simulink model "sampleModel1430"  (R2023a)
settings: Solver=VariableStepAuto  StartTime=0.0  StopTime=10.0  RelTol=1e-3
libraries: hdlsllib x6, simulink x2
settings Model: Creator=user1  LastModifiedBy=user1

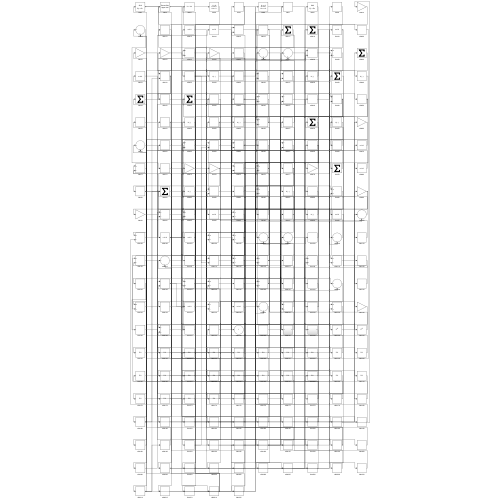
[thumbnail: Simulink's stored preview of the top-level diagram]
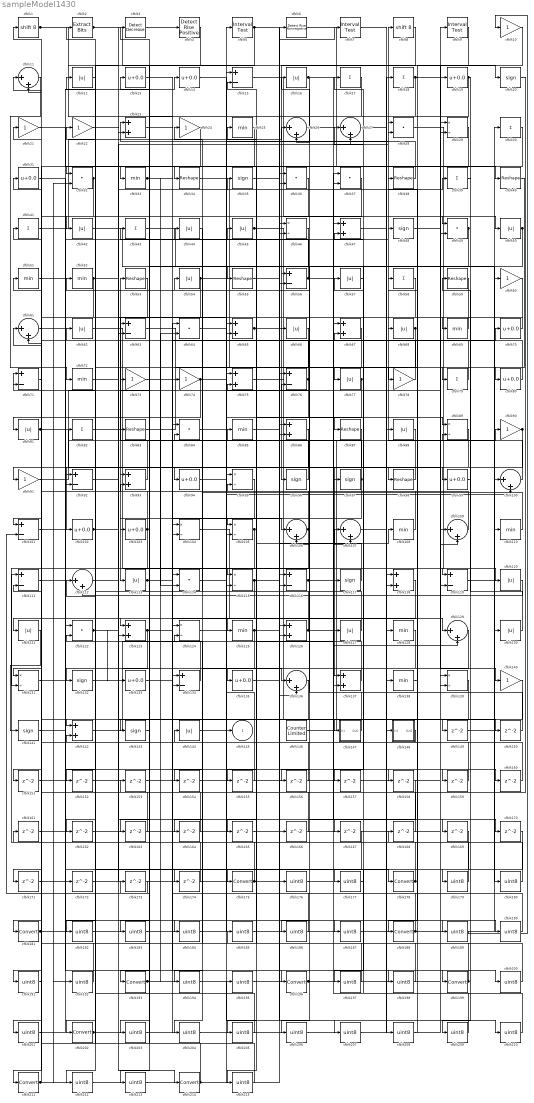
== system sampleModel1430 ==
  cfblk1 : ArithShift  BitShiftNumber=8
  cfblk{10,21..22,24,60,73..74,78,90..91,140} (11 alike) : Gain
  cfblk{11,26..27,61,100,106..107,109,112,129,136} (11 alike) : Sum  Inputs=|++
  cfblk{15,56,63,71,76,92,101,111,116,119,134} (11 alike) : Sum  Inputs=+-
  cfblk{13..14,19,31,70,80,94,99,102..103,133,135} (12 alike) : Bias  Bias=0.0  SaturateOnIntegerOverflow=off
  cfblk{29,46,89,95,104..105,115,124,131,139} (10 alike) : Product  Inputs=*/  RndMeth=Zero  SaturateOnIntegerOverflow=on
  cfblk{25,33,51..52,69,72,85,108,110,125,128,138} (12 alike) : MinMax
  cfblk{12,16,42,44..45,50,54,57,62,66,68,77,81,88,113,120..121,127,130,144} (20 alike) : Abs  SaturateOnIntegerOverflow=off
  cfblk{28,32,36..37,49,64,84,114,122} (9 alike) : DotProduct  OutDataTypeStr=Inherit: Inherit via internal rule
  cfblk{20,35,48,96..97,117,132,141,143} (9 alike) : Signum
  cfblk{23,47,65,67,75,86,93,118,123,126,137,142} (12 alike) : Sum
  cfblk146 : hdlsllib/Sources/Counter Limited  uplimit=7  tsamp=-1
  cfblk147 : Subsystem
      settings: LibrarySourceBlock=|
      | hdlsllib/Ports &
      | Subsystems/Subsystem
  cfblk148 : Subsystem
      settings: LibrarySourceBlock=|
      | hdlsllib/Ports &
      | Subsystems/Subsystem
  cfblk{149..174} (26 alike) : Delay  SampleTime=1
  cfblk{17..18,30,39,41,43,58,79,82} (9 alike) : Sum  Inputs=+
  cfblk{175,178,181,188,193,196,199,202,211,214} (10 alike) : DataTypeConversion  SaturateOnIntegerOverflow=off  RndMeth=Floor
  cfblk{176..177,179..180,182..187,189..192,194..195,197..198,200..201,203..210,212..213,215} (31 alike) : DataTypeConversion  OutDataTypeStr=uint8  SaturateOnIntegerOverflow=off  RndMeth=Floor
  cfblk2 : simulink/Logic and Bit Operations/Extract Bits  bitsToExtract=Upper half  numBits=8  bitIdxRange=[0 7]  outScalingMode=Preserve fixed-point scaling
      settings: LibrarySourceBlock=|
      | hdlsllib/Logic and Bit
      | Operations/Extract Bits
  cfblk3 : simulink/Logic and Bit Operations/Detect Decrease  vinit=0.0  OutDataTypeStr=boolean
      settings: LibrarySourceBlock=|
      | hdlsllib/Logic and Bit
      | Operations/Detect
      | Decrease
  cfblk{34,38,40,53,55,59,83,87,98} (9 alike) : Reshape
  cfblk4 : hdlsllib/Logic and Bit Operations/Detect Rise Positive  vinit=0  OutDataTypeStr=boolean
  cfblk5 : hdlsllib/Logic and Bit Operations/Interval Test  IntervalClosedRight=on  uplimit=0.5  IntervalClosedLeft=on  lowlimit=-0.5  OutDataTypeStr=boolean
  cfblk6 : hdlsllib/Logic and Bit Operations/Detect Rise Nonnegative  vinit=0  OutDataTypeStr=boolean
  cfblk7 : hdlsllib/Logic and Bit Operations/Interval Test  IntervalClosedRight=on  uplimit=0.5  IntervalClosedLeft=on  lowlimit=-0.5  OutDataTypeStr=boolean
  cfblk8 : ArithShift  BitShiftNumber=8
  cfblk9 : hdlsllib/Logic and Bit Operations/Interval Test  IntervalClosedRight=on  uplimit=0.5  IntervalClosedLeft=on  lowlimit=-0.5  OutDataTypeStr=boolean
  cfblk145 : Outport  VectorParamsAs1DForOutWhenUnconnected=off
  wires:
  cfblk146/1 -> cfblk90/1
  cfblk50/1 -> cfblk156/1, cfblk157/1
  cfblk25/1 -> cfblk34/1
  cfblk62/1 -> cfblk119/1
  cfblk75/1 -> cfblk147/1(In1)
  cfblk97/1 -> cfblk85/1, cfblk134/2
  cfblk83/1 -> cfblk77/1
  cfblk33/1 -> cfblk129/1, cfblk114/2, cfblk187/1
  cfblk28/1 -> cfblk120/1
  cfblk40/1 -> cfblk80/1
  cfblk130/1 -> cfblk59/1
  cfblk100/1 -> cfblk8/1
  cfblk123/1 -> cfblk142/1, cfblk89/2, cfblk150/1
  cfblk88/1 -> cfblk137/1
  cfblk45/1 -> cfblk98/1, cfblk28/2
  cfblk3/1 -> cfblk4/1
  cfblk102/1 -> cfblk27/2, cfblk76/2, cfblk184/1
  cfblk52/1 -> cfblk121/1, cfblk189/1
  cfblk8/1 -> cfblk96/1
  cfblk78/1 -> cfblk54/1
  cfblk15/1 -> cfblk50/1
  cfblk92/1 -> cfblk199/1
  cfblk104/1 -> cfblk127/1
  cfblk67/1 -> cfblk175/1
  cfblk93/1 -> cfblk53/1
  cfblk122/1 -> cfblk133/1, cfblk149/1
  cfblk139/1 -> cfblk202/1
  cfblk41/1 -> cfblk26/1
  cfblk82/1 -> cfblk113/1
  cfblk30/1 -> cfblk181/1
  cfblk11/1 -> cfblk72/1
  cfblk56/1 -> cfblk43/1, cfblk169/1
  cfblk114/1 -> cfblk5/1
  cfblk89/1 -> cfblk102/1
  cfblk49/1 -> cfblk105/1, cfblk137/2, cfblk56/1
  cfblk116/1 -> cfblk16/1, cfblk129/2
  cfblk79/1 -> cfblk31/1
  cfblk1/1 -> cfblk104/1, cfblk23/2
  cfblk98/1 -> cfblk94/1
  cfblk77/1 -> cfblk115/1, cfblk106/2
  cfblk34/1 -> cfblk110/1
  cfblk70/1 -> cfblk69/1
  cfblk138/1 -> cfblk38/1
  cfblk64/1 -> cfblk145/1
  cfblk59/1 -> cfblk93/1
  cfblk108/1 -> cfblk57/1
  cfblk134/1 -> cfblk62/1
  cfblk27/1 -> cfblk88/1
  cfblk19/1 -> cfblk103/1, cfblk99/1
  cfblk55/1 -> cfblk6/1
  cfblk54/1 -> cfblk203/1, cfblk210/1
  cfblk7/1 -> cfblk49/1
  cfblk147/1(Out1) -> cfblk52/1
  cfblk125/1 -> cfblk108/1, cfblk164/1
  cfblk9/1 -> cfblk119/2
  cfblk43/1 -> cfblk130/1
  cfblk111/1 -> cfblk178/1
  cfblk37/1 -> cfblk193/1
  cfblk103/1 -> cfblk51/1, cfblk151/1
  cfblk117/1 -> cfblk45/1
  cfblk94/1 -> cfblk28/1
  cfblk106/1 -> cfblk2/1, cfblk152/1
  cfblk10/1 -> cfblk188/1
  cfblk124/1 -> cfblk196/1
  cfblk42/1 -> cfblk109/1
  cfblk5/1 -> cfblk32/1, cfblk143/1, cfblk207/1
  cfblk126/1 -> cfblk24/1, cfblk107/2
  cfblk46/1 -> cfblk123/1
  cfblk22/1 -> cfblk214/1
  cfblk144/1 -> cfblk39/1
  cfblk91/1 -> cfblk9/1
  cfblk18/1 -> cfblk78/1, cfblk140/1, cfblk56/2
  cfblk65/1 -> cfblk148/1(In1), cfblk89/1
  cfblk2/1 -> cfblk20/1, cfblk65/2
  cfblk112/1 -> cfblk35/1
  cfblk6/1 -> cfblk138/1
  cfblk113/1 -> cfblk93/2, cfblk68/1
  cfblk142/1 -> cfblk117/1
  cfblk110/1 -> cfblk44/1
  cfblk51/1 -> cfblk48/1
  cfblk32/1 -> cfblk131/1, cfblk201/1
  cfblk137/1 -> cfblk15/2
  cfblk109/1 -> cfblk73/1
  cfblk81/1 -> cfblk109/2, cfblk84/2
  cfblk58/1 -> cfblk81/1
  cfblk38/1 -> cfblk23/1
  cfblk68/1 -> cfblk125/1, cfblk165/1
  cfblk115/1 -> cfblk107/1, cfblk171/1
  cfblk69/1 -> cfblk66/1
  cfblk84/1 -> cfblk87/1
  cfblk96/1 -> cfblk63/1
  cfblk86/1 -> cfblk211/1
  cfblk101/1 -> cfblk14/1
  cfblk90/1 -> cfblk135/1, cfblk123/2
  cfblk143/1 -> cfblk83/1
  cfblk36/1 -> cfblk42/1
  cfblk127/1 -> cfblk71/1
  cfblk121/1 -> cfblk141/1
  cfblk80/1 -> cfblk3/1
  cfblk13/1 -> cfblk126/2
  cfblk120/1 -> cfblk112/2
  cfblk4/1 -> cfblk33/1
  cfblk12/1 -> cfblk132/1
  cfblk63/1 -> cfblk128/1
  cfblk105/1 -> cfblk131/2, cfblk115/2
  cfblk132/1 -> cfblk136/1
  cfblk71/1 -> cfblk101/1
  cfblk29/1 -> cfblk55/1
  cfblk23/1 -> cfblk106/1
  cfblk57/1 -> cfblk17/1
  cfblk48/1 -> cfblk29/2
  cfblk35/1 -> cfblk7/1
  cfblk135/1 -> cfblk136/2
  cfblk76/1 -> cfblk116/2, cfblk11/1
  cfblk148/1(Out1) -> cfblk144/1
  cfblk16/1 -> cfblk26/2, cfblk79/1
  cfblk14/1 -> cfblk100/2
  cfblk21/1 -> cfblk40/1
  cfblk73/1 -> cfblk134/1
  cfblk74/1 -> cfblk91/1, cfblk70/1
  cfblk149/1 -> cfblk100/1
  cfblk150/1 -> cfblk75/1
  cfblk151/1 -> cfblk104/2
  cfblk152/1 -> cfblk29/1
  cfblk20/1 -> cfblk153/1
  cfblk153/1 -> cfblk105/2
  cfblk44/1 -> cfblk154/1
  cfblk87/1 -> cfblk155/1
  cfblk155/1 -> cfblk65/1
  cfblk156/1 -> cfblk15/1
  cfblk157/1 -> cfblk27/1
  cfblk26/1 -> cfblk158/1
  cfblk31/1 -> cfblk159/1
  cfblk159/1 -> cfblk126/1
  cfblk85/1 -> cfblk160/1
  cfblk160/1 -> cfblk1/1
  cfblk161/1 -> cfblk49/2
  cfblk53/1 -> cfblk162/1
  cfblk162/1 -> cfblk116/1
  cfblk17/1 -> cfblk163/1
  cfblk163/1 -> cfblk112/1
  cfblk164/1 -> cfblk71/2
  cfblk165/1 -> cfblk76/1
  cfblk166/1 -> cfblk142/2
  cfblk72/1 -> cfblk167/1
  cfblk168/1 -> cfblk122/1
  cfblk107/1 -> cfblk170/1
  cfblk171/1 -> cfblk46/2
  cfblk141/1 -> cfblk172/1
  cfblk172/1 -> cfblk63/2
  cfblk173/1 -> cfblk101/2
  cfblk136/1 -> cfblk174/1
  cfblk174/1 -> cfblk12/1
  cfblk175/1 -> cfblk21/1, cfblk114/1
  cfblk176/1 -> cfblk67/1
  cfblk154/1 -> cfblk177/1
  cfblk177/1 -> cfblk67/2
  cfblk178/1 -> cfblk84/1, cfblk25/1
  cfblk39/1 -> cfblk179/1
  cfblk179/1 -> cfblk111/1
  cfblk119/1 -> cfblk180/1
  cfblk180/1 -> cfblk111/2
  cfblk181/1 -> cfblk161/1, cfblk82/1, cfblk97/1
  cfblk66/1 -> cfblk182/1
  cfblk182/1 -> cfblk30/1
  cfblk95/1 -> cfblk183/1
  cfblk183/1 -> cfblk36/2
  cfblk184/1 -> cfblk95/1
  cfblk185/1 -> cfblk95/2
  cfblk60/1 -> cfblk186/1
  cfblk186/1 -> cfblk36/1
  cfblk187/1 -> cfblk60/1
  cfblk188/1 -> cfblk58/1, cfblk46/1
  cfblk189/1 -> cfblk10/1
  cfblk61/1 -> cfblk190/1
  cfblk190/1 -> cfblk64/1
  cfblk140/1 -> cfblk191/1
  cfblk191/1 -> cfblk61/1
  cfblk192/1 -> cfblk61/2
  cfblk193/1 -> cfblk176/1, cfblk64/2
  cfblk170/1 -> cfblk194/1
  cfblk194/1 -> cfblk37/1
  cfblk195/1 -> cfblk37/2
  cfblk196/1 -> cfblk18/1, cfblk19/1
  cfblk169/1 -> cfblk197/1
  cfblk197/1 -> cfblk124/1
  cfblk131/1 -> cfblk198/1
  cfblk198/1 -> cfblk124/2
  cfblk199/1 -> cfblk185/1, cfblk75/2
  cfblk133/1 -> cfblk200/1
  cfblk200/1 -> cfblk92/1
  cfblk201/1 -> cfblk92/2
  cfblk202/1 -> cfblk166/1, cfblk74/1
  cfblk203/1 -> cfblk139/1
  cfblk129/1 -> cfblk204/1
  cfblk204/1 -> cfblk139/2
  cfblk118/1 -> cfblk205/1
  cfblk205/1 -> cfblk122/2
  cfblk158/1 -> cfblk206/1
  cfblk206/1 -> cfblk118/1
  cfblk207/1 -> cfblk118/2
  cfblk47/1 -> cfblk208/1
  cfblk208/1 -> cfblk168/1
  cfblk99/1 -> cfblk209/1
  cfblk209/1 -> cfblk47/1
  cfblk210/1 -> cfblk47/2
  cfblk211/1 -> cfblk195/1, cfblk192/1, cfblk32/2, cfblk41/1
  cfblk167/1 -> cfblk212/1
  cfblk212/1 -> cfblk86/1
  cfblk24/1 -> cfblk213/1
  cfblk213/1 -> cfblk86/2
  cfblk214/1 -> cfblk173/1, cfblk11/2, cfblk13/1
  cfblk128/1 -> cfblk215/1
  cfblk215/1 -> cfblk22/1

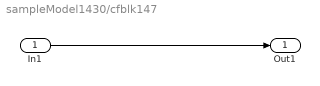
== system sampleModel1430/cfblk147 ==
  In1 : Inport
  Out1 : Outport
  wires:
  In1/1 -> Out1/1

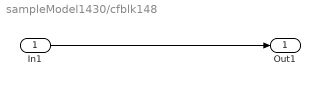
== system sampleModel1430/cfblk148 ==
  In1 : Inport
  Out1 : Outport
  wires:
  In1/1 -> Out1/1
